simulink model "IRB140_speed"  (R2019a)
settings: Solver=VariableStepAuto  StartTime=0.0  StopTime=10.0  RelTol=1e-3
InitFcn:
  | rpm_max=5000;
  | trq_stall=7;
  | T_i=1e-3;
  | eta=100;
  | rpm_eta=3000;
  | trq_eta=2.07;
  | J=0.672*1e-4;
  | rpm0=0;
  | gearRatio=10;
  | ts=0.0025;
undefined symbols (not defined in the file or in its folder): sigbuilder_block, X, Y, Z
libraries: sm_lib x61, fl_lib x37, nesl_utility x31, simulink x12, eeGeneralControl x12, ee_lib x6
(part 3 of 3)

== system IRB140_speed/Plant/robot/link_6 ==
  Inertia : sm_lib/Body Elements/Inertia  InertiaType=Custom  Mass=0.0258654328719498  MassUnits=kg  CenterOfMass=[0, 0, 0]  CenterOfMassUnits=m  MomentsOfInertia=[5.9822143548355e-06, 6.2921914507958e-06, 6.17479327327778e-06]  MomentsOfInertiaUnits=kg*m^2  ProductsOfInertia=[6.75626369217644e-13, -3.33091906738059e-13, 4.58244484401765e-08]  ProductsOfInertiaUnits=kg*m^2  GraphicType=None  MarkerShape=Inertia  MarkerSize=20  GraphicVisPropType=SimpleVisualProperties  GraphicDiffuseColor=[0.5 0.5 0.5]  GraphicSpecularColor=[0.5 0.5 0.5 1.0]  GraphicAmbientColor=[0.15 0.15 0.15 1.0]  GraphicEmissiveColor=[0.0 0.0 0.0 1.0]  GraphicShininess=75  GraphicOpacity=1.0
  InertiaOriginTransform : sm_lib/Frames and Transforms/Rigid Transform  TranslationMethod=Cartesian  TranslationStandardOffset=0  TranslationLengthUnit=m  TranslationStandardAxis=+Z  TranslationCartesianOffset=[0.502059432845099, -0.711774967143511, 2.38785136319277e-10]  TranslationROffset=0  TranslationROffsetUnits=m  TranslationZOffset=0  TranslationZOffsetUnits=m  TranslationThetaOffset=0  TranslationThetaOffsetUnits=deg  RotationMethod=RotationSequence  RotationAngleUnits=deg  RotationStandardAxis=+Z  RotationAngle=0.0  RotationArbitraryAxis=[0 0 1]  FollAlignAxisA=+X  BaseAlignAxisA=+Y  FollAlignAxisB=+Y  BaseAlignAxisB=+Z  RotationSequenceAxes=BaseAxes  RotationSequence=XYZ  RotationSequenceAngles=[0, 0, 0]  RotationSequenceAnglesUnits=rad  RotationMatrix=[1 0 0; 0 1 0; 0 0 1]
  ReferenceFrame : sm_lib/Frames and Transforms/Reference Frame
  Visual : sm_lib/Body Elements/Solid  InertiaType=Custom  Mass=0  MassUnits=kg  CenterOfMass=[0, 0, 0]  CenterOfMassUnits=m  MomentsOfInertia=[0, 0, 0]  MomentsOfInertiaUnits=kg*m^2  ProductsOfInertia=[0, 0, 0]  ProductsOfInertiaUnits=kg*m^2  BasedOnType=Density  Density=1000  DensityUnits=kg/m^3  DoExposeReferenceFrame=on  SerializedFrames=<Frames/>  GraphicType=FromGeometry  MarkerShape=Sphere  MarkerSize=10  GraphicVisPropType=SimpleVisualProperties  GraphicDiffuseColor=[0.796078431372549, 0.823529411764706, 0.937254901960784]  GraphicSpecularColor=[0.5 0.5 0.5 1.0]  GraphicAmbientColor=[0.15 0.15 0.15 1.0]  GraphicEmissiveColor=[0.0 0.0 0.0 1.0]  GraphicShininess=75  GraphicOpacity=1  GeometryShape=FromFile  RectangleSize=[1 1]  RectangleSizeUnits=m  BrickDimensions=[1 1 1]  BrickDimensionUnits=m  CylinderRadius=1  CylinderRadiusUnits=m  CylinderLength=1  CylinderLengthUnits=m  SphereRadius=1  SphereRadiusUnits=m  EllipsoidRadii=[1 1 1]  EllipsoidRadiiUnits=m  ExtrusionCrossSection=[1 1; -1 1; -1 -1; 1 -1]  ExtrusionCrossSectionUnits=m  ExtrusionLength=1  ExtrusionLengthUnits=m  PolygonNumSides=3  PolygonOuterRadius=1  PolygonOuterRadiusUnits=m  ExtGeomFileType=STL  ExtGeomFileName=IRB140/urdf/meshes/link6.stl  ExtGeomFileUnits=m  RevolutionCrossSection=[1 1; 1 -1; 2 -1; 2 1]  RevolutionCrossSectionUnits=m  RevolutionExtent=Full  RevolutionAngle=180  RevolutionAngleUnits=deg
  VisualOriginTransform : sm_lib/Frames and Transforms/Rigid Transform  TranslationMethod=Cartesian  TranslationStandardOffset=0  TranslationLengthUnit=m  TranslationStandardAxis=+Z  TranslationCartesianOffset=[-0.515, 0.712, 0]  TranslationROffset=0  TranslationROffsetUnits=m  TranslationZOffset=0  TranslationZOffsetUnits=m  TranslationThetaOffset=0  TranslationThetaOffsetUnits=deg  RotationMethod=RotationSequence  RotationAngleUnits=deg  RotationStandardAxis=+Z  RotationAngle=0.0  RotationArbitraryAxis=[0 0 1]  FollAlignAxisA=+X  BaseAlignAxisA=+Y  FollAlignAxisB=+Y  BaseAlignAxisB=+Z  RotationSequenceAxes=BaseAxes  RotationSequence=XYZ  RotationSequenceAngles=[0, 0, 0]  RotationSequenceAnglesUnits=rad  RotationMatrix=[1 0 0; 0 1 0; 0 0 1]
  joint6_AxisInvTransform : sm_lib/Frames and Transforms/Rigid Transform  TranslationMethod=Cartesian  TranslationStandardOffset=0  TranslationLengthUnit=m  TranslationStandardAxis=+Z  TranslationCartesianOffset=[0, 0, 0]  TranslationROffset=0  TranslationROffsetUnits=m  TranslationZOffset=0  TranslationZOffsetUnits=m  TranslationThetaOffset=0  TranslationThetaOffsetUnits=deg  RotationMethod=ArbitraryAxis  RotationAngleUnits=rad  RotationStandardAxis=+Z  RotationAngle=1.570796326794897  RotationArbitraryAxis=[-0, 1, 0]  FollAlignAxisA=+X  BaseAlignAxisA=+Y  FollAlignAxisB=+Y  BaseAlignAxisB=+Z  RotationSequenceAxes=FollowerAxes  RotationSequence=XYX  RotationSequenceAngles=[0 0 0]  RotationSequenceAnglesUnits=deg  RotationMatrix=[1 0 0; 0 1 0; 0 0 1]
  F : PMIOPort  Side=Left
  connections:
  Inertia/RConn1 -- InertiaOriginTransform/RConn1
  ReferenceFrame/RConn1 -- InertiaOriginTransform/LConn1 -- VisualOriginTransform/LConn1 -- joint6_AxisInvTransform/LConn1
  Visual/RConn1 -- VisualOriginTransform/RConn1
  joint6_AxisInvTransform/RConn1 -- F/RConn1

== system IRB140_speed/Plant/servo system/Subsystem1 ==
  torqueCommand : Inport
  Subsystem : Subsystem
  + : PMIOPort  Side=Left
  - : PMIOPort  Port=2  Side=Left
  R1 : PMIOPort  Port=3  Side=Right
  C1 : PMIOPort  Port=4  Side=Right
  torque1 : Outport
  motVel1 : Outport  Port=2  Unit=rpm
  wires:
  Subsystem/1(torque) -> torque1/1
  Subsystem/2(motVel) -> motVel1/1
  torqueCommand/1 -> Subsystem/1(torqueCommand)
  connections:
  Subsystem/RConn2 -- C1/RConn1
  Subsystem/LConn2 -- -/RConn1
  Subsystem/LConn1 -- +/RConn1
  Subsystem/RConn1 -- R1/RConn1

== system IRB140_speed/Plant/servo system/Subsystem2 ==
  torqueCommand : Inport
  Subsystem : Subsystem
  + : PMIOPort  Side=Left
  - : PMIOPort  Port=2  Side=Left
  R1 : PMIOPort  Port=3  Side=Right
  C1 : PMIOPort  Port=4  Side=Right
  torque1 : Outport
  motVel1 : Outport  Port=2  Unit=rpm
  wires:
  Subsystem/1(torque) -> torque1/1
  Subsystem/2(motVel) -> motVel1/1
  torqueCommand/1 -> Subsystem/1(torqueCommand)
  connections:
  Subsystem/RConn2 -- C1/RConn1
  Subsystem/LConn2 -- -/RConn1
  Subsystem/LConn1 -- +/RConn1
  Subsystem/RConn1 -- R1/RConn1

== system IRB140_speed/Plant/servo system/Subsystem3 ==
  torqueCommand : Inport
  Subsystem : Subsystem
  + : PMIOPort  Side=Left
  - : PMIOPort  Port=2  Side=Left
  R1 : PMIOPort  Port=3  Side=Right
  C1 : PMIOPort  Port=4  Side=Right
  torque1 : Outport
  motVel1 : Outport  Port=2  Unit=rpm
  wires:
  Subsystem/1(torque) -> torque1/1
  Subsystem/2(motVel) -> motVel1/1
  torqueCommand/1 -> Subsystem/1(torqueCommand)
  connections:
  Subsystem/RConn2 -- C1/RConn1
  Subsystem/LConn2 -- -/RConn1
  Subsystem/LConn1 -- +/RConn1
  Subsystem/RConn1 -- R1/RConn1

== system IRB140_speed/Plant/servo system/Subsystem4 ==
  torqueCommand : Inport
  Subsystem : Subsystem
  + : PMIOPort  Side=Left
  - : PMIOPort  Port=2  Side=Left
  R1 : PMIOPort  Port=3  Side=Right
  C1 : PMIOPort  Port=4  Side=Right
  torque1 : Outport
  motVel1 : Outport  Port=2  Unit=rpm
  wires:
  Subsystem/1(torque) -> torque1/1
  Subsystem/2(motVel) -> motVel1/1
  torqueCommand/1 -> Subsystem/1(torqueCommand)
  connections:
  Subsystem/RConn2 -- C1/RConn1
  Subsystem/LConn2 -- -/RConn1
  Subsystem/LConn1 -- +/RConn1
  Subsystem/RConn1 -- R1/RConn1

== system IRB140_speed/Plant/servo system/Subsystem5 ==
  torqueCommand : Inport
  Subsystem : Subsystem
  + : PMIOPort  Side=Left
  - : PMIOPort  Port=2  Side=Left
  R1 : PMIOPort  Port=3  Side=Right
  C1 : PMIOPort  Port=4  Side=Right
  torque1 : Outport
  motVel1 : Outport  Port=2  Unit=rpm
  wires:
  Subsystem/1(torque) -> torque1/1
  Subsystem/2(motVel) -> motVel1/1
  torqueCommand/1 -> Subsystem/1(torqueCommand)
  connections:
  Subsystem/RConn2 -- C1/RConn1
  Subsystem/LConn2 -- -/RConn1
  Subsystem/LConn1 -- +/RConn1
  Subsystem/RConn1 -- R1/RConn1

== system IRB140_speed/Plant/servo system/Subsystem6 ==
  torqueCommand : Inport
  Subsystem : Subsystem
  + : PMIOPort  Side=Left
  - : PMIOPort  Port=2  Side=Left
  R1 : PMIOPort  Port=3  Side=Right
  C1 : PMIOPort  Port=4  Side=Right
  torque1 : Outport
  motVel1 : Outport  Port=2  Unit=rpm
  wires:
  Subsystem/1(torque) -> torque1/1
  Subsystem/2(motVel) -> motVel1/1
  torqueCommand/1 -> Subsystem/1(torqueCommand)
  connections:
  Subsystem/RConn2 -- C1/RConn1
  Subsystem/LConn2 -- -/RConn1
  Subsystem/LConn1 -- +/RConn1
  Subsystem/RConn1 -- R1/RConn1

== system IRB140_speed/Plant/robot/Subsystem/rot2rev  ==
  Ideal Angular Velocity Source : fl_lib/Mechanical/Mechanical Sources/Ideal Angular Velocity Source
  Ideal Torque Sensor : fl_lib/Mechanical/Mechanical Sensors/Ideal Torque Sensor
  w : PMIOPort  Side=Right
  R : PMIOPort  Port=2  Side=Right
  t : PMIOPort  Port=3  Side=Left
  C : PMIOPort  Port=4  Side=Left
  connections:
  w/RConn1 -- Ideal Angular Velocity Source/RConn1
  Ideal Torque Sensor/RConn2 -- t/RConn1
  Ideal Angular Velocity Source/LConn1 -- R/RConn1
  C/RConn1 -- Ideal Torque Sensor/RConn1
  Ideal Torque Sensor/LConn1 -- Ideal Angular Velocity Source/RConn2

== system IRB140_speed/Plant/robot/Subsystem1/rot2rev  ==
  Ideal Angular Velocity Source : fl_lib/Mechanical/Mechanical Sources/Ideal Angular Velocity Source
  Ideal Torque Sensor : fl_lib/Mechanical/Mechanical Sensors/Ideal Torque Sensor
  w : PMIOPort  Side=Right
  R : PMIOPort  Port=2  Side=Right
  t : PMIOPort  Port=3  Side=Left
  C : PMIOPort  Port=4  Side=Left
  connections:
  w/RConn1 -- Ideal Angular Velocity Source/RConn1
  Ideal Torque Sensor/RConn2 -- t/RConn1
  Ideal Angular Velocity Source/LConn1 -- R/RConn1
  C/RConn1 -- Ideal Torque Sensor/RConn1
  Ideal Torque Sensor/LConn1 -- Ideal Angular Velocity Source/RConn2

== system IRB140_speed/Plant/robot/Subsystem2/rot2rev  ==
  Ideal Angular Velocity Source : fl_lib/Mechanical/Mechanical Sources/Ideal Angular Velocity Source
  Ideal Torque Sensor : fl_lib/Mechanical/Mechanical Sensors/Ideal Torque Sensor
  w : PMIOPort  Side=Right
  R : PMIOPort  Port=2  Side=Right
  t : PMIOPort  Port=3  Side=Left
  C : PMIOPort  Port=4  Side=Left
  connections:
  w/RConn1 -- Ideal Angular Velocity Source/RConn1
  Ideal Torque Sensor/RConn2 -- t/RConn1
  Ideal Angular Velocity Source/LConn1 -- R/RConn1
  C/RConn1 -- Ideal Torque Sensor/RConn1
  Ideal Torque Sensor/LConn1 -- Ideal Angular Velocity Source/RConn2

== system IRB140_speed/Plant/robot/Subsystem3/rot2rev  ==
  Ideal Angular Velocity Source : fl_lib/Mechanical/Mechanical Sources/Ideal Angular Velocity Source
  Ideal Torque Sensor : fl_lib/Mechanical/Mechanical Sensors/Ideal Torque Sensor
  w : PMIOPort  Side=Right
  R : PMIOPort  Port=2  Side=Right
  t : PMIOPort  Port=3  Side=Left
  C : PMIOPort  Port=4  Side=Left
  connections:
  w/RConn1 -- Ideal Angular Velocity Source/RConn1
  Ideal Torque Sensor/RConn2 -- t/RConn1
  Ideal Angular Velocity Source/LConn1 -- R/RConn1
  C/RConn1 -- Ideal Torque Sensor/RConn1
  Ideal Torque Sensor/LConn1 -- Ideal Angular Velocity Source/RConn2

== system IRB140_speed/Plant/robot/Subsystem4/rot2rev  ==
  Ideal Angular Velocity Source : fl_lib/Mechanical/Mechanical Sources/Ideal Angular Velocity Source
  Ideal Torque Sensor : fl_lib/Mechanical/Mechanical Sensors/Ideal Torque Sensor
  w : PMIOPort  Side=Right
  R : PMIOPort  Port=2  Side=Right
  t : PMIOPort  Port=3  Side=Left
  C : PMIOPort  Port=4  Side=Left
  connections:
  w/RConn1 -- Ideal Angular Velocity Source/RConn1
  Ideal Torque Sensor/RConn2 -- t/RConn1
  Ideal Angular Velocity Source/LConn1 -- R/RConn1
  C/RConn1 -- Ideal Torque Sensor/RConn1
  Ideal Torque Sensor/LConn1 -- Ideal Angular Velocity Source/RConn2

== system IRB140_speed/Plant/robot/Subsystem5/rot2rev  ==
  Ideal Angular Velocity Source : fl_lib/Mechanical/Mechanical Sources/Ideal Angular Velocity Source
  Ideal Torque Sensor : fl_lib/Mechanical/Mechanical Sensors/Ideal Torque Sensor
  w : PMIOPort  Side=Right
  R : PMIOPort  Port=2  Side=Right
  t : PMIOPort  Port=3  Side=Left
  C : PMIOPort  Port=4  Side=Left
  connections:
  w/RConn1 -- Ideal Angular Velocity Source/RConn1
  Ideal Torque Sensor/RConn2 -- t/RConn1
  Ideal Angular Velocity Source/LConn1 -- R/RConn1
  C/RConn1 -- Ideal Torque Sensor/RConn1
  Ideal Torque Sensor/LConn1 -- Ideal Angular Velocity Source/RConn2

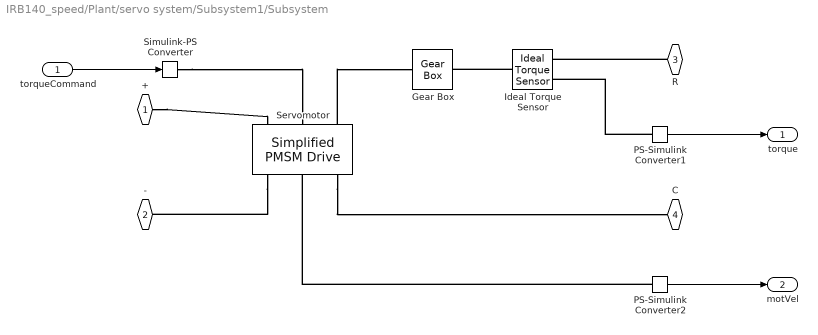
== system IRB140_speed/Plant/servo system/Subsystem1/Subsystem ==
  torqueCommand : Inport
  Gear Box : fl_lib/Mechanical/Mechanisms/Gear Box  ratio=gearRatio  t_in_specify=off  t_in_priority=None  t_in=0 N*m  t_in_nominal_specify=off  t_in_nominal_unit=N*m  t_in_nominal_value=1  t_out_specify=off  t_out_priority=None  t_out=0 N*m  t_out_nominal_specify=off  t_out_nominal_unit=N*m  t_out_nominal_value=1
  Ideal Torque Sensor : fl_lib/Mechanical/Mechanical Sensors/Ideal Torque Sensor
  PS-Simulink Converter1 : nesl_utility/PS-Simulink Converter  PhysicalDomain=network_engine_domain  SubClassName=ps_output  LeftPortType=input  RightPortType=output  PseudoPeriodic=off  Frequencies=[]  Unit=N*m  AffineConversion=off
  PS-Simulink Converter2 : nesl_utility/PS-Simulink Converter  PhysicalDomain=network_engine_domain  SubClassName=ps_output  LeftPortType=input  RightPortType=output  PseudoPeriodic=off  Frequencies=[]  Unit=rpm  AffineConversion=off
  Servomotor : ee_lib/Electromechanical/Permanent Magnet/Simplified PMSM Drive  torque_speed_param=1  w_t=[0 0.98 0.99 1] * rpm_max rpm  T_t=[1 1 1 0] * trq_stall N*m  torque_max=0.1 N*m  power_max=30 W  Tc=T_i s  losses_param=1  eff=eta  w_eff=rpm_eta rpm  T_eff=trq_eta N*m  Piron=0 W  Pbase=0 W  w_eff_vec=[-8000 -4000 0 4000 8000] rpm  T_eff_vec=[0 0.03 0.06 0.09] N*m  v_eff_vec=[100, 250, 400] V  losses_mat=[1.49 1.67 2.21 3.10; 0.42 0.69 1.14 2.03; 0.06 0.24 0.78 1.68; 0.42 0.69 1.14 2.03; 1.49 1.67 2.21 3.10] W  efficiency_mat=[95 95 95 95; 95 95 95 95; 95 95 95 95; 95 95 95 95; 95 95 95 95]  losses_mat_3D=ones(5, 4, 3) W  efficiency_mat_3D=95 * ones(5, 4, 3)  Res=0 Ohm  J=J kg*m^2  lam=0 N*m/(rad/s)  speed0=rpm0 rpm  faulted_specify=off  faulted_priority=None  faulted=0  faulted_nominal_specify=off  faulted_nominal_unit=1  faulted_nominal_value=1  alpha=3.93e-3 1/K  Tmeas=25 degC  Tmeas2=125 degC  losses_mat_T2=[1.49, 1.74, 2.49, 3.74; .42, .67, 1.42, 2.67; .06, .31, 1.06, 2.31; .42, .67, 1.42, 2.67; 1.49, 1.74, 2.49, 3.74] W  efficiency_mat_T2=[95, 95, 95, 95; 95, 95, 95, 95; 95, 95, 95, 95; 95, 95, 95, 95; 95, 95, 95, 95]  losses_mat_3D_T2=ones(5, 4, 3) W  efficiency_mat_3D_T2=95 * ones(5, 4, 3)  thermal_mass=100 J/K  initial_temperature=25 degC  fault_condition=1  fault_threshold=0.5
      settings: SourceProductName=Simscape Electrical  SourceProductBaseCode=PS
  Simulink-PS Converter : nesl_utility/Simulink-PS Converter  PhysicalDomain=network_engine_domain  SubClassName=ps_input  LeftPortType=input  RightPortType=output  PseudoPeriodic=off  Frequencies=[]  NoiseDistribution=none  NoiseParameters=[]  Unit=N*m  AffineConversion=off  FilteringAndDerivatives=filter  SimscapeFilterOrder=2  InputFilterTimeConstant=0.001  UdotUserProvided=0
  + : PMIOPort  Side=Left
  - : PMIOPort  Port=2  Side=Left
  R : PMIOPort  Port=3  Side=Right
  C : PMIOPort  Port=4  Side=Right
  torque : Outport
  motVel : Outport  Port=2  Unit=rpm
  wires:
  PS-Simulink Converter1/1 -> torque/1
  torqueCommand/1 -> Simulink-PS Converter/1
  PS-Simulink Converter2/1 -> motVel/1
  connections:
  Simulink-PS Converter/RConn1 -- Servomotor/LConn2
  R/RConn1 -- Ideal Torque Sensor/RConn1
  Servomotor/LConn3 -- Gear Box/LConn1
  PS-Simulink Converter1/LConn1 -- Ideal Torque Sensor/RConn2
  Ideal Torque Sensor/LConn1 -- Gear Box/RConn1
  Servomotor/RConn1 -- -/RConn1
  +/RConn1 -- Servomotor/LConn1
  PS-Simulink Converter2/LConn1 -- Servomotor/RConn2
  Servomotor/RConn3 -- C/RConn1

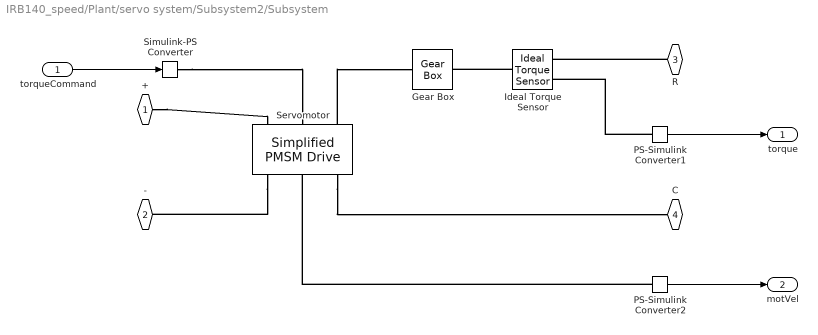
== system IRB140_speed/Plant/servo system/Subsystem2/Subsystem ==
  torqueCommand : Inport
  Gear Box : fl_lib/Mechanical/Mechanisms/Gear Box  ratio=gearRatio  t_in_specify=off  t_in_priority=None  t_in=0 N*m  t_in_nominal_specify=off  t_in_nominal_unit=N*m  t_in_nominal_value=1  t_out_specify=off  t_out_priority=None  t_out=0 N*m  t_out_nominal_specify=off  t_out_nominal_unit=N*m  t_out_nominal_value=1
  Ideal Torque Sensor : fl_lib/Mechanical/Mechanical Sensors/Ideal Torque Sensor
  PS-Simulink Converter1 : nesl_utility/PS-Simulink Converter  PhysicalDomain=network_engine_domain  SubClassName=ps_output  LeftPortType=input  RightPortType=output  PseudoPeriodic=off  Frequencies=[]  Unit=N*m  AffineConversion=off
  PS-Simulink Converter2 : nesl_utility/PS-Simulink Converter  PhysicalDomain=network_engine_domain  SubClassName=ps_output  LeftPortType=input  RightPortType=output  PseudoPeriodic=off  Frequencies=[]  Unit=rpm  AffineConversion=off
  Servomotor : ee_lib/Electromechanical/Permanent Magnet/Simplified PMSM Drive  torque_speed_param=1  w_t=[0 0.98 0.99 1] * rpm_max rpm  T_t=[1 1 1 0] * trq_stall N*m  torque_max=0.1 N*m  power_max=30 W  Tc=T_i s  losses_param=1  eff=eta  w_eff=rpm_eta rpm  T_eff=trq_eta N*m  Piron=0 W  Pbase=0 W  w_eff_vec=[-8000 -4000 0 4000 8000] rpm  T_eff_vec=[0 0.03 0.06 0.09] N*m  v_eff_vec=[100, 250, 400] V  losses_mat=[1.49 1.67 2.21 3.10; 0.42 0.69 1.14 2.03; 0.06 0.24 0.78 1.68; 0.42 0.69 1.14 2.03; 1.49 1.67 2.21 3.10] W  efficiency_mat=[95 95 95 95; 95 95 95 95; 95 95 95 95; 95 95 95 95; 95 95 95 95]  losses_mat_3D=ones(5, 4, 3) W  efficiency_mat_3D=95 * ones(5, 4, 3)  Res=0 Ohm  J=J kg*m^2  lam=0 N*m/(rad/s)  speed0=rpm0 rpm  faulted_specify=off  faulted_priority=None  faulted=0  faulted_nominal_specify=off  faulted_nominal_unit=1  faulted_nominal_value=1  alpha=3.93e-3 1/K  Tmeas=25 degC  Tmeas2=125 degC  losses_mat_T2=[1.49, 1.74, 2.49, 3.74; .42, .67, 1.42, 2.67; .06, .31, 1.06, 2.31; .42, .67, 1.42, 2.67; 1.49, 1.74, 2.49, 3.74] W  efficiency_mat_T2=[95, 95, 95, 95; 95, 95, 95, 95; 95, 95, 95, 95; 95, 95, 95, 95; 95, 95, 95, 95]  losses_mat_3D_T2=ones(5, 4, 3) W  efficiency_mat_3D_T2=95 * ones(5, 4, 3)  thermal_mass=100 J/K  initial_temperature=25 degC  fault_condition=1  fault_threshold=0.5
      settings: SourceProductName=Simscape Electrical  SourceProductBaseCode=PS
  Simulink-PS Converter : nesl_utility/Simulink-PS Converter  PhysicalDomain=network_engine_domain  SubClassName=ps_input  LeftPortType=input  RightPortType=output  PseudoPeriodic=off  Frequencies=[]  NoiseDistribution=none  NoiseParameters=[]  Unit=N*m  AffineConversion=off  FilteringAndDerivatives=filter  SimscapeFilterOrder=2  InputFilterTimeConstant=0.001  UdotUserProvided=0
  + : PMIOPort  Side=Left
  - : PMIOPort  Port=2  Side=Left
  R : PMIOPort  Port=3  Side=Right
  C : PMIOPort  Port=4  Side=Right
  torque : Outport
  motVel : Outport  Port=2  Unit=rpm
  wires:
  PS-Simulink Converter1/1 -> torque/1
  torqueCommand/1 -> Simulink-PS Converter/1
  PS-Simulink Converter2/1 -> motVel/1
  connections:
  Simulink-PS Converter/RConn1 -- Servomotor/LConn2
  R/RConn1 -- Ideal Torque Sensor/RConn1
  Servomotor/LConn3 -- Gear Box/LConn1
  PS-Simulink Converter1/LConn1 -- Ideal Torque Sensor/RConn2
  Ideal Torque Sensor/LConn1 -- Gear Box/RConn1
  Servomotor/RConn1 -- -/RConn1
  +/RConn1 -- Servomotor/LConn1
  PS-Simulink Converter2/LConn1 -- Servomotor/RConn2
  Servomotor/RConn3 -- C/RConn1

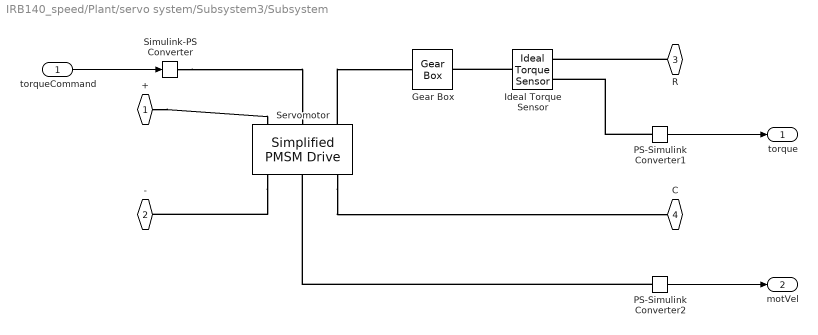
== system IRB140_speed/Plant/servo system/Subsystem3/Subsystem ==
  torqueCommand : Inport
  Gear Box : fl_lib/Mechanical/Mechanisms/Gear Box  ratio=gearRatio  t_in_specify=off  t_in_priority=None  t_in=0 N*m  t_in_nominal_specify=off  t_in_nominal_unit=N*m  t_in_nominal_value=1  t_out_specify=off  t_out_priority=None  t_out=0 N*m  t_out_nominal_specify=off  t_out_nominal_unit=N*m  t_out_nominal_value=1
  Ideal Torque Sensor : fl_lib/Mechanical/Mechanical Sensors/Ideal Torque Sensor
  PS-Simulink Converter1 : nesl_utility/PS-Simulink Converter  PhysicalDomain=network_engine_domain  SubClassName=ps_output  LeftPortType=input  RightPortType=output  PseudoPeriodic=off  Frequencies=[]  Unit=N*m  AffineConversion=off
  PS-Simulink Converter2 : nesl_utility/PS-Simulink Converter  PhysicalDomain=network_engine_domain  SubClassName=ps_output  LeftPortType=input  RightPortType=output  PseudoPeriodic=off  Frequencies=[]  Unit=rpm  AffineConversion=off
  Servomotor : ee_lib/Electromechanical/Permanent Magnet/Simplified PMSM Drive  torque_speed_param=1  w_t=[0 0.98 0.99 1] * rpm_max rpm  T_t=[1 1 1 0] * trq_stall N*m  torque_max=0.1 N*m  power_max=30 W  Tc=T_i s  losses_param=1  eff=eta  w_eff=rpm_eta rpm  T_eff=trq_eta N*m  Piron=0 W  Pbase=0 W  w_eff_vec=[-8000 -4000 0 4000 8000] rpm  T_eff_vec=[0 0.03 0.06 0.09] N*m  v_eff_vec=[100, 250, 400] V  losses_mat=[1.49 1.67 2.21 3.10; 0.42 0.69 1.14 2.03; 0.06 0.24 0.78 1.68; 0.42 0.69 1.14 2.03; 1.49 1.67 2.21 3.10] W  efficiency_mat=[95 95 95 95; 95 95 95 95; 95 95 95 95; 95 95 95 95; 95 95 95 95]  losses_mat_3D=ones(5, 4, 3) W  efficiency_mat_3D=95 * ones(5, 4, 3)  Res=0 Ohm  J=J kg*m^2  lam=0 N*m/(rad/s)  speed0=rpm0 rpm  faulted_specify=off  faulted_priority=None  faulted=0  faulted_nominal_specify=off  faulted_nominal_unit=1  faulted_nominal_value=1  alpha=3.93e-3 1/K  Tmeas=25 degC  Tmeas2=125 degC  losses_mat_T2=[1.49, 1.74, 2.49, 3.74; .42, .67, 1.42, 2.67; .06, .31, 1.06, 2.31; .42, .67, 1.42, 2.67; 1.49, 1.74, 2.49, 3.74] W  efficiency_mat_T2=[95, 95, 95, 95; 95, 95, 95, 95; 95, 95, 95, 95; 95, 95, 95, 95; 95, 95, 95, 95]  losses_mat_3D_T2=ones(5, 4, 3) W  efficiency_mat_3D_T2=95 * ones(5, 4, 3)  thermal_mass=100 J/K  initial_temperature=25 degC  fault_condition=1  fault_threshold=0.5
      settings: SourceProductName=Simscape Electrical  SourceProductBaseCode=PS
  Simulink-PS Converter : nesl_utility/Simulink-PS Converter  PhysicalDomain=network_engine_domain  SubClassName=ps_input  LeftPortType=input  RightPortType=output  PseudoPeriodic=off  Frequencies=[]  NoiseDistribution=none  NoiseParameters=[]  Unit=N*m  AffineConversion=off  FilteringAndDerivatives=filter  SimscapeFilterOrder=2  InputFilterTimeConstant=0.001  UdotUserProvided=0
  + : PMIOPort  Side=Left
  - : PMIOPort  Port=2  Side=Left
  R : PMIOPort  Port=3  Side=Right
  C : PMIOPort  Port=4  Side=Right
  torque : Outport
  motVel : Outport  Port=2  Unit=rpm
  wires:
  PS-Simulink Converter1/1 -> torque/1
  torqueCommand/1 -> Simulink-PS Converter/1
  PS-Simulink Converter2/1 -> motVel/1
  connections:
  Simulink-PS Converter/RConn1 -- Servomotor/LConn2
  R/RConn1 -- Ideal Torque Sensor/RConn1
  Servomotor/LConn3 -- Gear Box/LConn1
  PS-Simulink Converter1/LConn1 -- Ideal Torque Sensor/RConn2
  Ideal Torque Sensor/LConn1 -- Gear Box/RConn1
  Servomotor/RConn1 -- -/RConn1
  +/RConn1 -- Servomotor/LConn1
  PS-Simulink Converter2/LConn1 -- Servomotor/RConn2
  Servomotor/RConn3 -- C/RConn1

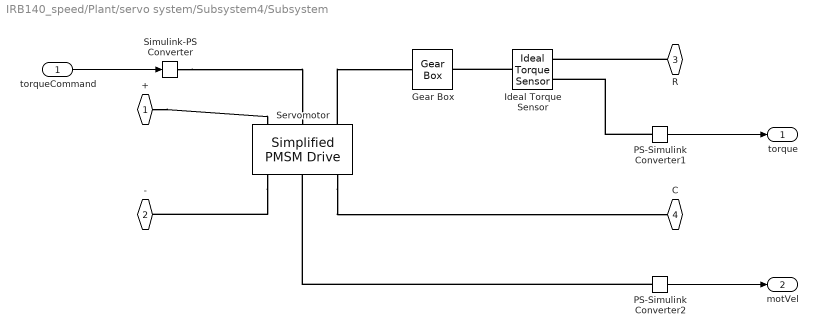
== system IRB140_speed/Plant/servo system/Subsystem4/Subsystem ==
  torqueCommand : Inport
  Gear Box : fl_lib/Mechanical/Mechanisms/Gear Box  ratio=gearRatio  t_in_specify=off  t_in_priority=None  t_in=0 N*m  t_in_nominal_specify=off  t_in_nominal_unit=N*m  t_in_nominal_value=1  t_out_specify=off  t_out_priority=None  t_out=0 N*m  t_out_nominal_specify=off  t_out_nominal_unit=N*m  t_out_nominal_value=1
  Ideal Torque Sensor : fl_lib/Mechanical/Mechanical Sensors/Ideal Torque Sensor
  PS-Simulink Converter1 : nesl_utility/PS-Simulink Converter  PhysicalDomain=network_engine_domain  SubClassName=ps_output  LeftPortType=input  RightPortType=output  PseudoPeriodic=off  Frequencies=[]  Unit=N*m  AffineConversion=off
  PS-Simulink Converter2 : nesl_utility/PS-Simulink Converter  PhysicalDomain=network_engine_domain  SubClassName=ps_output  LeftPortType=input  RightPortType=output  PseudoPeriodic=off  Frequencies=[]  Unit=rpm  AffineConversion=off
  Servomotor : ee_lib/Electromechanical/Permanent Magnet/Simplified PMSM Drive  torque_speed_param=1  w_t=[0 0.98 0.99 1] * rpm_max rpm  T_t=[1 1 1 0] * trq_stall N*m  torque_max=0.1 N*m  power_max=30 W  Tc=T_i s  losses_param=1  eff=eta  w_eff=rpm_eta rpm  T_eff=trq_eta N*m  Piron=0 W  Pbase=0 W  w_eff_vec=[-8000 -4000 0 4000 8000] rpm  T_eff_vec=[0 0.03 0.06 0.09] N*m  v_eff_vec=[100, 250, 400] V  losses_mat=[1.49 1.67 2.21 3.10; 0.42 0.69 1.14 2.03; 0.06 0.24 0.78 1.68; 0.42 0.69 1.14 2.03; 1.49 1.67 2.21 3.10] W  efficiency_mat=[95 95 95 95; 95 95 95 95; 95 95 95 95; 95 95 95 95; 95 95 95 95]  losses_mat_3D=ones(5, 4, 3) W  efficiency_mat_3D=95 * ones(5, 4, 3)  Res=0 Ohm  J=J kg*m^2  lam=0 N*m/(rad/s)  speed0=rpm0 rpm  faulted_specify=off  faulted_priority=None  faulted=0  faulted_nominal_specify=off  faulted_nominal_unit=1  faulted_nominal_value=1  alpha=3.93e-3 1/K  Tmeas=25 degC  Tmeas2=125 degC  losses_mat_T2=[1.49, 1.74, 2.49, 3.74; .42, .67, 1.42, 2.67; .06, .31, 1.06, 2.31; .42, .67, 1.42, 2.67; 1.49, 1.74, 2.49, 3.74] W  efficiency_mat_T2=[95, 95, 95, 95; 95, 95, 95, 95; 95, 95, 95, 95; 95, 95, 95, 95; 95, 95, 95, 95]  losses_mat_3D_T2=ones(5, 4, 3) W  efficiency_mat_3D_T2=95 * ones(5, 4, 3)  thermal_mass=100 J/K  initial_temperature=25 degC  fault_condition=1  fault_threshold=0.5
      settings: SourceProductName=Simscape Electrical  SourceProductBaseCode=PS
  Simulink-PS Converter : nesl_utility/Simulink-PS Converter  PhysicalDomain=network_engine_domain  SubClassName=ps_input  LeftPortType=input  RightPortType=output  PseudoPeriodic=off  Frequencies=[]  NoiseDistribution=none  NoiseParameters=[]  Unit=N*m  AffineConversion=off  FilteringAndDerivatives=filter  SimscapeFilterOrder=2  InputFilterTimeConstant=0.001  UdotUserProvided=0
  + : PMIOPort  Side=Left
  - : PMIOPort  Port=2  Side=Left
  R : PMIOPort  Port=3  Side=Right
  C : PMIOPort  Port=4  Side=Right
  torque : Outport
  motVel : Outport  Port=2  Unit=rpm
  wires:
  PS-Simulink Converter1/1 -> torque/1
  torqueCommand/1 -> Simulink-PS Converter/1
  PS-Simulink Converter2/1 -> motVel/1
  connections:
  Simulink-PS Converter/RConn1 -- Servomotor/LConn2
  R/RConn1 -- Ideal Torque Sensor/RConn1
  Servomotor/LConn3 -- Gear Box/LConn1
  PS-Simulink Converter1/LConn1 -- Ideal Torque Sensor/RConn2
  Ideal Torque Sensor/LConn1 -- Gear Box/RConn1
  Servomotor/RConn1 -- -/RConn1
  +/RConn1 -- Servomotor/LConn1
  PS-Simulink Converter2/LConn1 -- Servomotor/RConn2
  Servomotor/RConn3 -- C/RConn1

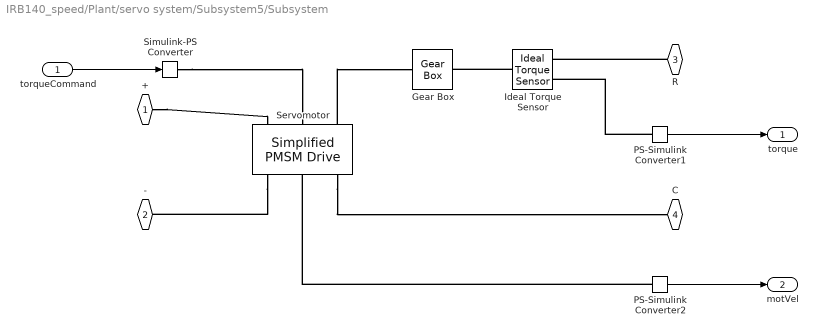
== system IRB140_speed/Plant/servo system/Subsystem5/Subsystem ==
  torqueCommand : Inport
  Gear Box : fl_lib/Mechanical/Mechanisms/Gear Box  ratio=gearRatio  t_in_specify=off  t_in_priority=None  t_in=0 N*m  t_in_nominal_specify=off  t_in_nominal_unit=N*m  t_in_nominal_value=1  t_out_specify=off  t_out_priority=None  t_out=0 N*m  t_out_nominal_specify=off  t_out_nominal_unit=N*m  t_out_nominal_value=1
  Ideal Torque Sensor : fl_lib/Mechanical/Mechanical Sensors/Ideal Torque Sensor
  PS-Simulink Converter1 : nesl_utility/PS-Simulink Converter  PhysicalDomain=network_engine_domain  SubClassName=ps_output  LeftPortType=input  RightPortType=output  PseudoPeriodic=off  Frequencies=[]  Unit=N*m  AffineConversion=off
  PS-Simulink Converter2 : nesl_utility/PS-Simulink Converter  PhysicalDomain=network_engine_domain  SubClassName=ps_output  LeftPortType=input  RightPortType=output  PseudoPeriodic=off  Frequencies=[]  Unit=rpm  AffineConversion=off
  Servomotor : ee_lib/Electromechanical/Permanent Magnet/Simplified PMSM Drive  torque_speed_param=1  w_t=[0 0.98 0.99 1] * rpm_max rpm  T_t=[1 1 1 0] * trq_stall N*m  torque_max=0.1 N*m  power_max=30 W  Tc=T_i s  losses_param=1  eff=eta  w_eff=rpm_eta rpm  T_eff=trq_eta N*m  Piron=0 W  Pbase=0 W  w_eff_vec=[-8000 -4000 0 4000 8000] rpm  T_eff_vec=[0 0.03 0.06 0.09] N*m  v_eff_vec=[100, 250, 400] V  losses_mat=[1.49 1.67 2.21 3.10; 0.42 0.69 1.14 2.03; 0.06 0.24 0.78 1.68; 0.42 0.69 1.14 2.03; 1.49 1.67 2.21 3.10] W  efficiency_mat=[95 95 95 95; 95 95 95 95; 95 95 95 95; 95 95 95 95; 95 95 95 95]  losses_mat_3D=ones(5, 4, 3) W  efficiency_mat_3D=95 * ones(5, 4, 3)  Res=0 Ohm  J=J kg*m^2  lam=0 N*m/(rad/s)  speed0=rpm0 rpm  faulted_specify=off  faulted_priority=None  faulted=0  faulted_nominal_specify=off  faulted_nominal_unit=1  faulted_nominal_value=1  alpha=3.93e-3 1/K  Tmeas=25 degC  Tmeas2=125 degC  losses_mat_T2=[1.49, 1.74, 2.49, 3.74; .42, .67, 1.42, 2.67; .06, .31, 1.06, 2.31; .42, .67, 1.42, 2.67; 1.49, 1.74, 2.49, 3.74] W  efficiency_mat_T2=[95, 95, 95, 95; 95, 95, 95, 95; 95, 95, 95, 95; 95, 95, 95, 95; 95, 95, 95, 95]  losses_mat_3D_T2=ones(5, 4, 3) W  efficiency_mat_3D_T2=95 * ones(5, 4, 3)  thermal_mass=100 J/K  initial_temperature=25 degC  fault_condition=1  fault_threshold=0.5
      settings: SourceProductName=Simscape Electrical  SourceProductBaseCode=PS
  Simulink-PS Converter : nesl_utility/Simulink-PS Converter  PhysicalDomain=network_engine_domain  SubClassName=ps_input  LeftPortType=input  RightPortType=output  PseudoPeriodic=off  Frequencies=[]  NoiseDistribution=none  NoiseParameters=[]  Unit=N*m  AffineConversion=off  FilteringAndDerivatives=filter  SimscapeFilterOrder=2  InputFilterTimeConstant=0.001  UdotUserProvided=0
  + : PMIOPort  Side=Left
  - : PMIOPort  Port=2  Side=Left
  R : PMIOPort  Port=3  Side=Right
  C : PMIOPort  Port=4  Side=Right
  torque : Outport
  motVel : Outport  Port=2  Unit=rpm
  wires:
  PS-Simulink Converter1/1 -> torque/1
  torqueCommand/1 -> Simulink-PS Converter/1
  PS-Simulink Converter2/1 -> motVel/1
  connections:
  Simulink-PS Converter/RConn1 -- Servomotor/LConn2
  R/RConn1 -- Ideal Torque Sensor/RConn1
  Servomotor/LConn3 -- Gear Box/LConn1
  PS-Simulink Converter1/LConn1 -- Ideal Torque Sensor/RConn2
  Ideal Torque Sensor/LConn1 -- Gear Box/RConn1
  Servomotor/RConn1 -- -/RConn1
  +/RConn1 -- Servomotor/LConn1
  PS-Simulink Converter2/LConn1 -- Servomotor/RConn2
  Servomotor/RConn3 -- C/RConn1

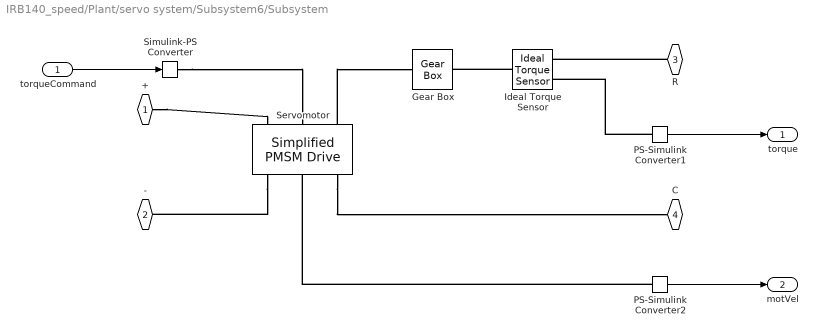
== system IRB140_speed/Plant/servo system/Subsystem6/Subsystem ==
  torqueCommand : Inport
  Gear Box : fl_lib/Mechanical/Mechanisms/Gear Box  ratio=gearRatio  t_in_specify=off  t_in_priority=None  t_in=0 N*m  t_in_nominal_specify=off  t_in_nominal_unit=N*m  t_in_nominal_value=1  t_out_specify=off  t_out_priority=None  t_out=0 N*m  t_out_nominal_specify=off  t_out_nominal_unit=N*m  t_out_nominal_value=1
  Ideal Torque Sensor : fl_lib/Mechanical/Mechanical Sensors/Ideal Torque Sensor
  PS-Simulink Converter1 : nesl_utility/PS-Simulink Converter  PhysicalDomain=network_engine_domain  SubClassName=ps_output  LeftPortType=input  RightPortType=output  PseudoPeriodic=off  Frequencies=[]  Unit=N*m  AffineConversion=off
  PS-Simulink Converter2 : nesl_utility/PS-Simulink Converter  PhysicalDomain=network_engine_domain  SubClassName=ps_output  LeftPortType=input  RightPortType=output  PseudoPeriodic=off  Frequencies=[]  Unit=rpm  AffineConversion=off
  Servomotor : ee_lib/Electromechanical/Permanent Magnet/Simplified PMSM Drive  torque_speed_param=1  w_t=[0 0.98 0.99 1] * rpm_max rpm  T_t=[1 1 1 0] * trq_stall N*m  torque_max=0.1 N*m  power_max=30 W  Tc=T_i s  losses_param=1  eff=eta  w_eff=rpm_eta rpm  T_eff=trq_eta N*m  Piron=0 W  Pbase=0 W  w_eff_vec=[-8000 -4000 0 4000 8000] rpm  T_eff_vec=[0 0.03 0.06 0.09] N*m  v_eff_vec=[100, 250, 400] V  losses_mat=[1.49 1.67 2.21 3.10; 0.42 0.69 1.14 2.03; 0.06 0.24 0.78 1.68; 0.42 0.69 1.14 2.03; 1.49 1.67 2.21 3.10] W  efficiency_mat=[95 95 95 95; 95 95 95 95; 95 95 95 95; 95 95 95 95; 95 95 95 95]  losses_mat_3D=ones(5, 4, 3) W  efficiency_mat_3D=95 * ones(5, 4, 3)  Res=0 Ohm  J=J kg*m^2  lam=0 N*m/(rad/s)  speed0=rpm0 rpm  faulted_specify=off  faulted_priority=None  faulted=0  faulted_nominal_specify=off  faulted_nominal_unit=1  faulted_nominal_value=1  alpha=3.93e-3 1/K  Tmeas=25 degC  Tmeas2=125 degC  losses_mat_T2=[1.49, 1.74, 2.49, 3.74; .42, .67, 1.42, 2.67; .06, .31, 1.06, 2.31; .42, .67, 1.42, 2.67; 1.49, 1.74, 2.49, 3.74] W  efficiency_mat_T2=[95, 95, 95, 95; 95, 95, 95, 95; 95, 95, 95, 95; 95, 95, 95, 95; 95, 95, 95, 95]  losses_mat_3D_T2=ones(5, 4, 3) W  efficiency_mat_3D_T2=95 * ones(5, 4, 3)  thermal_mass=100 J/K  initial_temperature=25 degC  fault_condition=1  fault_threshold=0.5
      settings: SourceProductName=Simscape Electrical  SourceProductBaseCode=PS
  Simulink-PS Converter : nesl_utility/Simulink-PS Converter  PhysicalDomain=network_engine_domain  SubClassName=ps_input  LeftPortType=input  RightPortType=output  PseudoPeriodic=off  Frequencies=[]  NoiseDistribution=none  NoiseParameters=[]  Unit=N*m  AffineConversion=off  FilteringAndDerivatives=filter  SimscapeFilterOrder=2  InputFilterTimeConstant=0.001  UdotUserProvided=0
  + : PMIOPort  Side=Left
  - : PMIOPort  Port=2  Side=Left
  R : PMIOPort  Port=3  Side=Right
  C : PMIOPort  Port=4  Side=Right
  torque : Outport
  motVel : Outport  Port=2  Unit=rpm
  wires:
  PS-Simulink Converter1/1 -> torque/1
  torqueCommand/1 -> Simulink-PS Converter/1
  PS-Simulink Converter2/1 -> motVel/1
  connections:
  Simulink-PS Converter/RConn1 -- Servomotor/LConn2
  R/RConn1 -- Ideal Torque Sensor/RConn1
  Servomotor/LConn3 -- Gear Box/LConn1
  PS-Simulink Converter1/LConn1 -- Ideal Torque Sensor/RConn2
  Ideal Torque Sensor/LConn1 -- Gear Box/RConn1
  Servomotor/RConn1 -- -/RConn1
  +/RConn1 -- Servomotor/LConn1
  PS-Simulink Converter2/LConn1 -- Servomotor/RConn2
  Servomotor/RConn3 -- C/RConn1

== matlab function IRB140_speed/Jacobian Function ==
  data: q1 input; P output; q2 input; q3 input; q4 input; q5 input; q6 input; e output; J output; Jv output; Jw output; G output
% Embedded Matlab Function for Jacobian Calculation
function [P, e, J,Jv,Jw,G]  = fcn(q1,q2,q3,q4,q5,q6)
% DH Parameters of the robot with joint initial condition
% d = [0.4 0 0 0.62 0 0.115]; a = [0.18 0.6 0.12 0 0 0];
% th = [th1 th2 th3 th4 th5 th6]; al = [pi/2 0 pi/2 pi/2 -pi/2 0];
th1=q1;
th2=q2;
th3=q3;
th4=q4;
th5=q5;
th6=q6;
d = [0 0.3521 0 -0.0001 0.0146 -0.0000];
a = [0 0.0700 0.3600 0.0001 0.3796 0];
th = [th1 th2 th3 th4 th5 th6]; 
al = [0 pi/2 0 -pi/2 pi/2 pi/2];

% Generalized transformation matrix for a link CS
% Tr = [cos(th) -sin(th)*cos(al)  sin(th)*sin(al) a*cos(th); ...
%       sin(th)  cos(th)*cos(al) -cos(th)*sin(al) a*sin(th); ...
%             0  sin(al)                  cos(al)         d; ...
%             0        0                       0          1]

%Forward kinematic transformation  matrices for individual link
A1 = [cos(th(1))  -sin(th(1))*cos(al(1))  sin(th(1))*sin(al(1)) a(1)*cos(th(1)); ...
      sin(th(1))   cos(th(1))*cos(al(1)) -cos(th(1))*sin(al(1)) a(1)*sin(th(1)); ...
               0              sin(al(1))             cos(al(1))            d(1); ...
               0                       0                      0              1];
A2 = [cos(th(2))  -sin(th(2))*cos(al(2))  sin(th(2))*sin(al(2)) a(2)*cos(th(2)); ...
      sin(th(2))   cos(th(2))*cos(al(2)) -cos(th(2))*sin(al(2)) a(2)*sin(th(2)); ...
               0              sin(al(2))             cos(al(2))            d(2); ...
               0                       0                      0              1];
A3 = [cos(th(3))  -sin(th(3))*cos(al(3))  sin(th(3))*sin(al(3)) a(3)*cos(th(3)); ...
      sin(th(3))   cos(th(3))*cos(al(3)) -cos(th(3))*sin(al(3)) a(3)*sin(th(3)); ...
               0              sin(al(3))             cos(al(3))            d(3); ...
               0                       0                      0              1];
A4 = [cos(th(4))  -sin(th(4))*cos(al(4))  sin(th(4))*sin(al(4)) a(4)*cos(th(4)); ...
      sin(th(4))   cos(th(4))*cos(al(4)) -cos(th(4))*sin(al(4)) a(4)*sin(th(4)); ...
               0              sin(al(4))             cos(al(4))            d(4); ...
               0                       0                      0              1];
A5 = [cos(th(5))  -sin(th(5))*cos(al(5))  sin(th(5))*sin(al(5)) a(5)*cos(th(5)); ...
      sin(th(5))   cos(th(5))*cos(al(5)) -cos(th(5))*sin(al(5)) a(5)*sin(th(5)); ...
               0              sin(al(5))             cos(al(5))            d(5); ...
               0                       0                      0              1];
A6 = [cos(th(6))  -sin(th(6))*cos(al(6))  sin(th(6))*sin(al(6)) a(6)*cos(th(6)); ...
      sin(th(6))   cos(th(6))*cos(al(6)) -cos(th(6))*sin(al(6)) a(6)*sin(th(6)); ...
               0              sin(al(6))             cos(al(6))            d(6); ...
               0                       0                      0              1];

% Transformation matrices for each joint w.r.t. base
T1 = A1;
T12 = A1*A2;
T123 = A1*A2*A3;
T1234 = A1*A2*A3*A4;
T12345 = A1*A2*A3*A4*A5;
T123456 = A1*A2*A3*A4*A5*A6;

% End effector position
P = T123456(1:3,4);

% Extraction of e1, ... e6 (Vectors along the joint axes, w.r.t the base)
e1 = [0 0 1];
e2 = T1(1:3,3);
e3 = T12(1:3,3);
e4 = T123(1:3,3);
e5 = T1234(1:3,3);
e6 = T12345(1:3,3);

e = [e1(1) e1(2) e1(3) e2(1) e2(2) e2(3) e3(1) e3(2) e3(3)...
     e4(1) e4(2) e4(3) e5(1) e5(2) e5(3) e6(1) e6(2) e6(3)];
 
% Extraction of a1e, a2e, a3e, a4e, a5e, a6e
% (Vectors joining origin of link i to the end effector, w.r.t the base)
a1e = T123456(1:3,4);
a2e = T123456(1:3,4) - T1(1:3,4);
a3e = T123456(1:3,4) - T12(1:3,4);
a4e = T123456(1:3,4) - T123(1:3,4);
a5e = T123456(1:3,4) - T1234(1:3,4);
a6e = T123456(1:3,4) - T12345(1:3,4);
%% Calculation of Jacobian
Jv = [0 0 0 0 0 0; 0 0 0 0 0 0; 0 0 0 0 0 0];
Jv(1:3,1) = cross(e1,a1e);
Jv(1:3,2) = cross(e2,a2e);
Jv(1:3,3) = cross(e3,a3e);
Jv(1:3,4) = cross(e4,a4e);
Jv(1:3,5) = cross(e5,a5e);
Jv(1:3,6) = cross(e6,a6e); 
Jw = [0 0 0 0 0 0; 0 0 0 0 0 0; 0 0 0 0 0 0];
Jw(1:3,1) =e1;
Jw(1:3,2) =e2;
Jw(1:3,3) =e3;
Jw(1:3,4) =e4;
Jw(1:3,5) =e5;
Jw(1:3,6) =e6;
J=[Jv;Jw];
%gravity
g0=[0 0 -9.80665];
m1=12.409016159487;m2=16.287755696602;m3=7.58037424484438;m4=8.03072730997701;m5=1.7702548022269;m6=0.0258654328719498;
z0=[0 0 1];z1=T1(1:3,3);z2=T12(1:3,3);z3=T123(1:3,3);z4=T1234(1:3,3);z5=T12345(1:3,3);
p1=T1(1:3,4);p2=T12(1:3,4);p3=T123(1:3,4);p4=T1234(1:3,4);p5=T12345(1:3,4);p6=T123456(1:3,4);



Jl1p1=cross(z0,p1);
Jl2p1=cross(z0,p2);Jl2p2=cross(z1,(p2-p1));
Jl3p1=cross(z0,p3);Jl3p2=cross(z1,(p3-p1));Jl3p3=cross(z2,(p3-p2));
Jl4p1=cross(z0,p4);Jl4p2=cross(z1,(p4-p1));Jl4p3=cross(z2,(p4-p2));Jl4p4=cross(z3,(p4-p3));
Jl5p1=cross(z0,p5);Jl5p2=cross(z1,(p5-p1));Jl5p3=cross(z2,(p5-p2));Jl5p4=cross(z3,(p5-p3));Jl5p5=cross(z4,(p5-p4));
Jl6p1=cross(z0,p6);Jl6p2=cross(z1,(p6-p1));Jl6p3=cross(z2,(p6-p2));Jl6p4=cross(z3,(p6-p3));Jl6p5=cross(z4,(p6-p4));Jl6p6=cross(z5,(p6-p5));
g1=-(m1*g0*Jl1p1'+m2*g0*Jl2p1'+m3*g0*Jl3p1'+m4*g0*Jl4p1'+m5*g0*Jl5p1'+m6*g0*Jl6p1');
g2=-(m2*g0*Jl2p2+m3*g0*Jl3p2+m4*g0*Jl4p2+m5*g0*Jl5p2+m6*g0*Jl6p2);
g3=-(m3*g0*Jl3p3+m4*g0*Jl4p3+m5*g0*Jl5p3+m6*g0*Jl6p3);
g4=-(m4*g0*Jl4p4+m5*g0*Jl5p4+m6*g0*Jl6p4);
g5=-(m5*g0*Jl5p5+m6*g0*Jl6p5);
g6=-(m6*g0*Jl6p6);
G=[g1;g2;g3;g4;g5;g6];
